simulink library "MSP_FSW_lib"  (R2016b)
settings: Solver=VariableStepAuto  StartTime=0.0  StopTime=10.0  RelTol=1e-3
undefined symbols (not defined in the file): cmd_MT_fsw, fsw_params, omega_radps, sc_mode, sc_quat, states, target
libraries: bus_stubs_fsw x3, extended_kalman_filter_lib x1, actuator_processing x1, command_generation x1, gs_prediction_lib x1, mag_vec_lib x1, sgp4_lib_fsw x1, sun_vector_lib x1, time_coord_rotation_lib x1, mode_selection x1, target_generation_lib x1
settings Model: Creator=taylorreynolds  LastModifiedBy=Sean

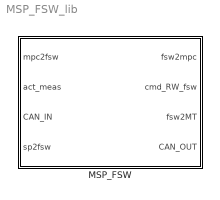
== system MSP_FSW_lib ==
  MSP_FSW : Subsystem

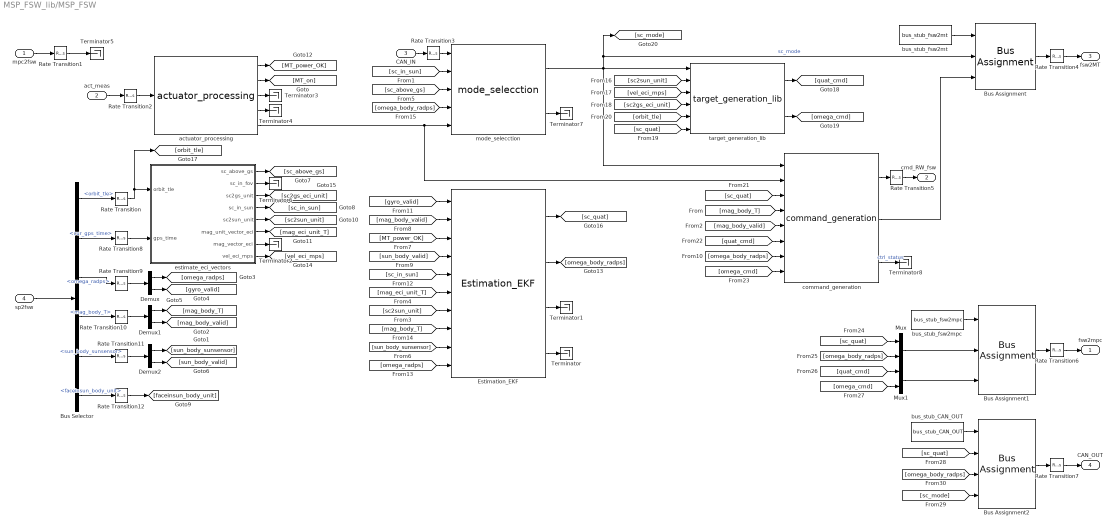
== system MSP_FSW_lib/MSP_FSW ==
  mpc2fsw : Inport  OutDataTypeStr=Bus: mpc2fsw
  act_meas : Inport  Port=2
  CAN_IN : Inport  Port=3  OutDataTypeStr=Bus: CAN_IN
  sp2fsw : Inport  Port=4  OutDataTypeStr=Bus: sp2fsw
  Bus Assignment : BusAssignment  AssignedSignals=sc_mode,cmd_MT_fsw
  Bus Assignment1 : BusAssignment  AssignedSignals=states,target
  Bus Assignment2 : BusAssignment  AssignedSignals=sc_quat,omega_radps,sc_mode
  Bus Selector : BusSelector  OutputSignals=orbit_tle,cur_gps_time,omega_radps,mag_body_T,sun_body_sunsensor,faceinsun_body_unit
  Demux : Demux  Outputs=[3 1]
  Demux1 : Demux  Outputs=[3 1]
  Demux2 : Demux  Outputs=[3 1]
  "Estimation_EKF " : extended_kalman_filter_lib/Estimation_EKF 
  Mux : Mux  Inputs=[4 3]
  Mux1 : Mux  Inputs=[4 3]
  Rate Transition : RateTransition  X0=fsw_params.environment.sgp4.orbit_tle  OutPortSampleTime=fsw_params.sample_time_s
  Rate Transition{1..3,9..12} (7 alike) : RateTransition  OutPortSampleTime=fsw_params.sample_time_s
  Rate Transition{4..7} (4 alike) : RateTransition
  Rate Transition8 : RateTransition  X0=fsw_params.sensor_processing.gps.ic.time  OutPortSampleTime=fsw_params.sample_time_s
  Terminator{,1..8} (9 alike) : Terminator
  actuator_processing : actuator_processing/actuator_processing
  bus_stub_CAN_OUT : bus_stubs_fsw/bus_stub_CAN_OUT
  bus_stub_fsw2mpc : bus_stubs_fsw/bus_stub_fsw2mpc
  bus_stub_fsw2mt : bus_stubs_fsw/bus_stub_fsw2mt
  command_generation : command_generation/command_generation
  estimate_eci_vectors : Subsystem
  mode_selecction : mode_selection/mode_selecction
  target_generation_lib : target_generation_lib/target_generation_lib
  fsw2mpc : Outport
  cmd_RW_fsw : Outport  Port=2
  fsw2MT : Outport  Port=3
  CAN_OUT : Outport  Port=4
  wires:
  [omega_body_radps] -> command_generation/7
  Rate Transition12/1 -> [faceinsun_body_unit]
  Rate Transition11/1 -> Demux2/1
  Rate Transition10/1 -> Demux1/1
  Rate Transition9/1 -> Demux/1
  Rate Transition8/1 -> estimate_eci_vectors/2(gps_time)
  Rate Transition/1 -> estimate_eci_vectors/1(orbit_tle), [orbit_tle]
  Bus Selector/1 -> Rate Transition/1  "<orbit_tle>"
  [sc_above_gs] -> mode_selecction/3
  estimate_eci_vectors/1(sc_above_gs) -> [sc_above_gs]
  "Estimation_EKF "/1 -> [sc_quat]
  command_generation/3 -> Terminator8/1  "ctrl_status"
  command_generation/2 -> Bus Assignment/3
  command_generation/1 -> Rate Transition5/1
  [mag_body_valid] -> command_generation/5
  [mag_body_T] -> command_generation/4
  [sc2sun_unit] -> "Estimation_EKF "/7
  [mag_eci_unit_T] -> "Estimation_EKF "/6
  [mag_body_T] -> "Estimation_EKF "/8
  [sun_body_sunsensor] -> "Estimation_EKF "/9
  [omega_radps] -> "Estimation_EKF "/10
  estimate_eci_vectors/3(sc2gs_unit) -> [sc2gs_eci_unit]
  estimate_eci_vectors/2(sc_in_fov) -> Terminator6/1
  estimate_eci_vectors/8(vel_eci_mps) -> [vel_eci_mps]
  actuator_processing/4 -> Terminator4/1
  actuator_processing/3 -> Terminator3/1
  CAN_IN/1 -> Rate Transition3/1
  estimate_eci_vectors/7(mag_vector_eci) -> Terminator2/1
  estimate_eci_vectors/6(mag_unit_vector_eci) -> [mag_eci_unit_T]
  estimate_eci_vectors/5(sc2sun_unit) -> [sc2sun_unit]
  "Estimation_EKF "/3 -> Terminator1/1
  "Estimation_EKF "/4 -> Terminator/1
  [sc_in_sun] -> "Estimation_EKF "/5
  [sun_body_valid] -> "Estimation_EKF "/4
  [MT_power_OK] -> "Estimation_EKF "/3
  estimate_eci_vectors/4(sc_in_sun) -> [sc_in_sun]
  [gyro_valid] -> "Estimation_EKF "/1
  [mag_body_valid] -> "Estimation_EKF "/2
  [sc_in_sun] -> mode_selecction/2
  mode_selecction/1 -> [sc_mode], Bus Assignment/2, command_generation/1, target_generation_lib/1  "sc_mode"
  Bus Selector/3 -> Rate Transition9/1  "<omega_radps>"
  Demux/1 -> [omega_radps]
  Demux/2 -> [gyro_valid]
  Bus Selector/4 -> Rate Transition10/1  "<mag_body_T>"
  Demux1/1 -> [mag_body_T]
  Demux1/2 -> [mag_body_valid]
  Bus Selector/5 -> Rate Transition11/1  "<sun_body_sunsensor>"
  Demux2/1 -> [sun_body_sunsensor]
  Demux2/2 -> [sun_body_valid]
  act_meas/1 -> Rate Transition2/1
  actuator_processing/1 -> [MT_power_OK]
  actuator_processing/2 -> [MT_on]
  Bus Selector/2 -> Rate Transition8/1  "<cur_gps_time>"
  "Estimation_EKF "/2 -> [omega_body_radps]
  actuator_processing/5 -> command_generation/2, mode_selecction/5
  [omega_body_radps] -> mode_selecction/4
  [sc2sun_unit] -> target_generation_lib/2
  [vel_eci_mps] -> target_generation_lib/3
  [sc2gs_eci_unit] -> target_generation_lib/4
  [sc_quat] -> target_generation_lib/6
  [orbit_tle] -> target_generation_lib/5
  [sc_quat] -> command_generation/3
  target_generation_lib/1 -> [quat_cmd]
  target_generation_lib/2 -> [omega_cmd]
  [quat_cmd] -> command_generation/6
  [omega_cmd] -> command_generation/8
  Bus Selector/6 -> Rate Transition12/1  "<faceinsun_body_unit>"
  mpc2fsw/1 -> Rate Transition1/1
  mode_selecction/2 -> Terminator7/1
  bus_stub_fsw2mt/1 -> Bus Assignment/1
  Bus Assignment/1 -> Rate Transition4/1
  Bus Assignment1/1 -> Rate Transition6/1
  bus_stub_fsw2mpc/1 -> Bus Assignment1/1
  [sc_quat] -> Mux/1
  [omega_body_radps] -> Mux/2
  Mux/1 -> Bus Assignment1/2
  [quat_cmd] -> Mux1/1
  [omega_cmd] -> Mux1/2
  Mux1/1 -> Bus Assignment1/3
  Bus Assignment2/1 -> Rate Transition7/1
  bus_stub_CAN_OUT/1 -> Bus Assignment2/1
  [sc_quat] -> Bus Assignment2/2
  [sc_mode] -> Bus Assignment2/4
  sp2fsw/1 -> Bus Selector/1
  Rate Transition1/1 -> Terminator5/1
  Rate Transition2/1 -> actuator_processing/1
  Rate Transition3/1 -> mode_selecction/1
  Rate Transition4/1 -> fsw2MT/1
  Rate Transition5/1 -> cmd_RW_fsw/1
  Rate Transition6/1 -> fsw2mpc/1
  Rate Transition7/1 -> CAN_OUT/1
  [omega_body_radps] -> Bus Assignment2/3

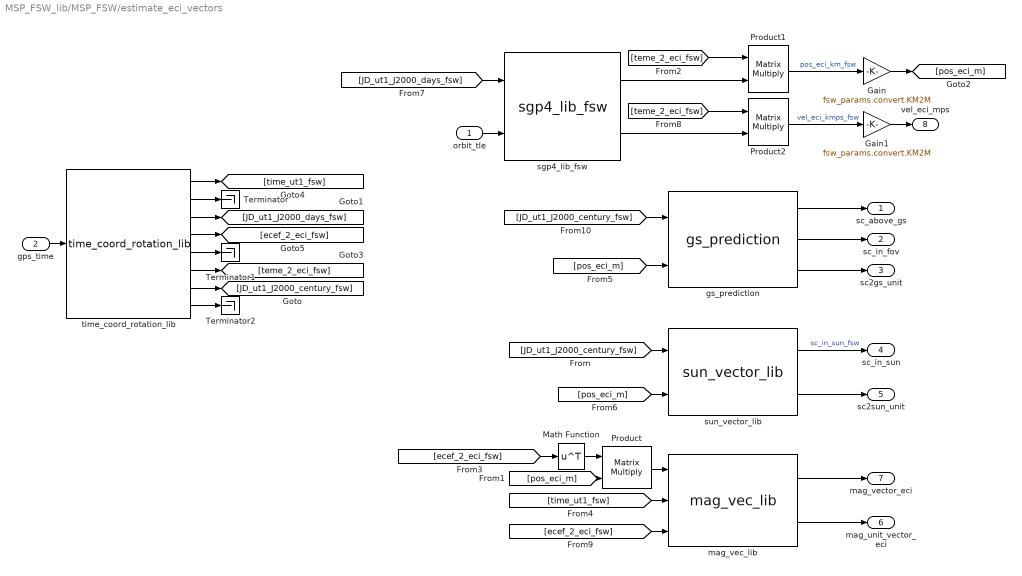
== system MSP_FSW_lib/MSP_FSW/estimate_eci_vectors ==
  orbit_tle : Inport
  gps_time : Inport  Port=2
  Gain : Gain  Gain=fsw_params.convert.KM2M
  Gain1 : Gain  Gain=fsw_params.convert.KM2M
  Math Function : Math  Operator=transpose  SaturateOnIntegerOverflow=on
  Product : Product  Multiplication=Matrix(*)
  Product1 : Product  Multiplication=Matrix(*)
  Product2 : Product  Multiplication=Matrix(*)
  Terminator : Terminator
  Terminator1 : Terminator
  Terminator2 : Terminator
  gs_prediction : gs_prediction_lib/gs_prediction
  mag_vec_lib : mag_vec_lib/mag_vec_lib
  sgp4_lib_fsw : sgp4_lib_fsw/sgp4_lib_fsw
  sun_vector_lib : sun_vector_lib/sun_vector_lib
  time_coord_rotation_lib : time_coord_rotation_lib/time_coord_rotation_lib
  sc_above_gs : Outport
  sc_in_fov : Outport  Port=2
  sc2gs_unit : Outport  Port=3
  sc_in_sun : Outport  Port=4
  sc2sun_unit : Outport  Port=5
  mag_unit_vector_eci : Outport  Port=6
  mag_vector_eci : Outport  Port=7
  vel_eci_mps : Outport  Port=8
  wires:
  mag_vec_lib/2 -> mag_unit_vector_eci/1
  mag_vec_lib/1 -> mag_vector_eci/1
  sun_vector_lib/2 -> sc2sun_unit/1
  [teme_2_eci_fsw] -> Product1/1
  [teme_2_eci_fsw] -> Product2/1
  [ecef_2_eci_fsw] -> Math Function/1
  [JD_ut1_J2000_century_fsw] -> sun_vector_lib/1
  [JD_ut1_J2000_days_fsw] -> sgp4_lib_fsw/1
  [ecef_2_eci_fsw] -> mag_vec_lib/3
  [time_ut1_fsw] -> mag_vec_lib/2
  sun_vector_lib/1 -> sc_in_sun/1  "sc_in_sun_fsw"
  Product2/1 -> Gain1/1  "vel_eci_kmps_fsw"
  sgp4_lib_fsw/2 -> Product2/2
  sgp4_lib_fsw/1 -> Product1/2
  Product1/1 -> Gain/1  "pos_eci_km_fsw"
  [pos_eci_m] -> Product/2
  [pos_eci_m] -> sun_vector_lib/2
  Gain1/1 -> vel_eci_mps/1
  Math Function/1 -> Product/1
  Product/1 -> mag_vec_lib/1
  Gain/1 -> [pos_eci_m]
  orbit_tle/1 -> sgp4_lib_fsw/2
  gps_time/1 -> time_coord_rotation_lib/1
  time_coord_rotation_lib/2 -> Terminator/1
  time_coord_rotation_lib/4 -> [ecef_2_eci_fsw]
  time_coord_rotation_lib/6 -> [teme_2_eci_fsw]
  time_coord_rotation_lib/1 -> [time_ut1_fsw]
  time_coord_rotation_lib/3 -> [JD_ut1_J2000_days_fsw]
  time_coord_rotation_lib/7 -> [JD_ut1_J2000_century_fsw]
  [pos_eci_m] -> gs_prediction/2
  [JD_ut1_J2000_century_fsw] -> gs_prediction/1
  gs_prediction/1 -> sc_above_gs/1
  gs_prediction/3 -> sc2gs_unit/1
  gs_prediction/2 -> sc_in_fov/1
  time_coord_rotation_lib/5 -> Terminator1/1
  time_coord_rotation_lib/8 -> Terminator2/1
